simulink model "MotorDrive_ShuntCapacitance_ProposedMethod2"  (R2018b)
settings: Solver=FixedStepAuto  StartTime=0.0  StopTime=10  RelTol=1e-3
libraries: powerlib x6, powerlib_meascontrol x5
settings Model: Creator=fkara  LastModifiedBy=nss

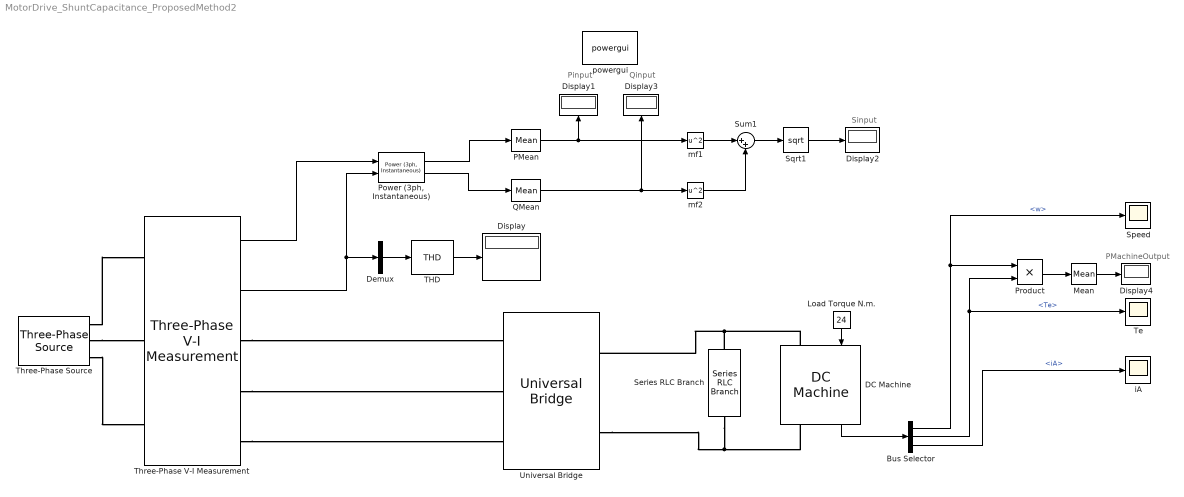
== system MotorDrive_ShuntCapacitance_ProposedMethod2 ==
  note: Pinput
  note: Qinput
  note: Sinput
  note: PMachineOutput
  Bus Selector : BusSelector  OutputSignals=w,Te,iA
  DC Machine : powerlib/Machines/DC Machine  PresetModel=No  MechanicalLoad=Torque TL  FieldType=Permanent magnet  ShowDetailedParameters=on  MeasurementBus=on  RLa="[10  0.01]"  RLf="[300  156]"  Laf=2  MachineConstant=Back-emf constant (V/rpm)  Ke=0.3  Kt=1.8  J=0.4  Bm=0  Tf=0  w0=1  Ifinit=1  TsPowergui=0  TsBlock=-1
  Demux : Demux  Outputs=1
  Display{,1..4} (5 alike) : Display
  Load Torque N.m. : Constant  Value=24
  Mean : powerlib_meascontrol/Measurements/Mean  Freq=60  Vinit=0  Ts=0
  PMean : powerlib_meascontrol/Measurements/Mean  Freq=60  Vinit=0  Ts=0
  "Power (3ph, Instantaneous)" : powerlib_meascontrol/Measurements/Power (3ph, Instantaneous)
      settings: SourceProductName=Simscape Power Systems
  Product : Product
  QMean : powerlib_meascontrol/Measurements/Mean  Freq=60  Vinit=0  Ts=0
  Series RLC Branch : powerlib/Elements/Series RLC Branch  LConnTagsString=__new0  RConnTagsString=__new0  BranchType=C  Resistance=1  Inductance=1e-3  SetiL0=off  InitialCurrent=0  Capacitance=0.1  Setx0=off  InitialVoltage=0  Measurements=None
  Speed : Scope
  Sqrt1 : Sqrt  SaturateOnIntegerOverflow=on
  Sum1 : Sum  Inputs=|++
  THD : powerlib_meascontrol/Measurements/THD  Freq=50  Ts=0
  Te : Scope
  Three-Phase V-I Measurement : powerlib/Measurements/Three-Phase V-I Measurement  VoltageMeasurement=phase-to-ground  SetLabelV=off  LabelV=Vabc  Vpu=off  VpuLL=off  CurrentMeasurement=yes  SetLabelI=off  LabelI=Iabc  Ipu=off  Pbase=100e6  Vbase=500e3  OutputType=Complex  PhasorSimulation=off  PSBequivalent=0
  Three-Phase Source : powerlib/Electrical Sources/Three-Phase Source  InternalConnection=Yg  VoltagePhases=off  Voltage=400  PhaseAngle=0  Voltage_phases=[25e3 25e3 25e3]/sqrt(3)  PhaseAngles_phases=[0 -120 +120]  Frequency=50  NonIdealSource=on  SpecifyImpedance=off  Resistance=100e-3  Inductance=100e-6  ShortCircuitLevel=100e6  BaseVoltage=400  XRratio=7  BusType=swing  Pref=10e3  Qref=0  Prefabc=[10e3, 10e3, 10e3]  Qrefabc=[0, 0, 0]  Qmin=-inf  Qmax=inf
  Universal Bridge : powerlib/Power Electronics/Universal Bridge  Arms=3  SnubberResistance=1e5  SnubberCapacitance=inf  Device=Diodes  Ron=20e-3  Lon=0  ForwardVoltages="[  0  0  ]"  ForwardVoltage=0.8  GTOparameters=[ 10e-6 , 20e-6 ]  IGBTparameters=[ 1e-6 , 2e-6 ]  Measurements=None  Measurements_2=None  converterType=Rectifier
  iA : Scope
  mf1 : Math  Operator=square  SaturateOnIntegerOverflow=on
  mf2 : Math  Operator=square  SaturateOnIntegerOverflow=on
  powergui : powerlib/powergui  Priority=1  SimulationMode=Discrete  SampleTime=50e-7  frequency=60  Iterations=50  frequencyindice=0  Pbase=100e6  ErrMax=1e-4  UnitsV=kV  UnitsW=MW  buscounter=0  FunctionMessages=off  echomessages=off  EnableUseOfTLC=off  CurrentSourceSwitches=off  DisableSnubberDevices=off  DisableRonSwitches=off  DisableVfSwitches=off  DisplayEquations=off  SolverType=Tustin/Backward Euler (TBE)  Interpol=off  ExternalGateDelay=off  methode=off  Ts=100  x0status=blocks  SPID=off  SwTol=0  HookPort=off  RestoreLinks=warning  ResistiveCurrentMeasurement=off  Frange=[0:2:500]  Ylog=off  Xlog=on  ShowGrid=off  save=off  variable=ZData  structure=0  ZoomFFT=off  StartTime=0.0  cycles=1  DisplayStyle=1  fundamental=60  FreqAxis=off  MaxFrequency=1000  frequencyindicesteady=1  RmsSteady=1  display=off
  wires:
  "Power (3ph, Instantaneous)"/1 -> PMean/1
  DC Machine/1 -> Bus Selector/1
  Product/1 -> Mean/1
  THD/1 -> Display/1
  mf1/1 -> Sum1/1
  Three-Phase V-I Measurement/1 -> "Power (3ph, Instantaneous)"/1
  Sum1/1 -> Sqrt1/1
  Mean/1 -> Display4/1
  PMean/1 -> mf1/1, Display1/1
  Demux/1 -> THD/1
  Sqrt1/1 -> Display2/1
  Bus Selector/2 -> Product/2, Te/1  "<Te>"
  Load Torque N.m./1 -> DC Machine/1
  Bus Selector/3 -> iA/1  "<iA>"
  mf2/1 -> Sum1/2
  Bus Selector/1 -> Speed/1, Product/1  "<w>"
  QMean/1 -> mf2/1, Display3/1
  Three-Phase V-I Measurement/2 -> Demux/1, "Power (3ph, Instantaneous)"/2
  "Power (3ph, Instantaneous)"/2 -> QMean/1
  connections:
  DC Machine/LConn1 -- Series RLC Branch/LConn1 -- Universal Bridge/RConn1
  Universal Bridge/RConn2 -- DC Machine/RConn1 -- Series RLC Branch/RConn1
  Three-Phase V-I Measurement/RConn1 -- Universal Bridge/LConn1
  Three-Phase Source/RConn3 -- Three-Phase V-I Measurement/LConn3
  Three-Phase Source/RConn2 -- Three-Phase V-I Measurement/LConn2
  Three-Phase V-I Measurement/RConn2 -- Universal Bridge/LConn2
  Three-Phase Source/RConn1 -- Three-Phase V-I Measurement/LConn1
  Three-Phase V-I Measurement/RConn3 -- Universal Bridge/LConn3
